simulink model "lab_2"  (R2017a)
settings: Solver=ode23tb  StartTime=0.0  StopTime=10.0  RelTol=1e-3
values from neighbouring files (symbols this model uses):
  c = 0.05    [K_Gain_matrix.m]    (also in Stepper_Model_2017_10_31_Script.m = 0.017; Stepper_Model_2017_Mark_Script.m)
  g = 9.82    [Stepper_Model_2017_10_31_Script.m]    (also in Stepper_Model_2017_Mark_Script.m)
  m = 0.2    [K_Gain_matrix.m]    (also in Stepper_Model_2017_10_31_Script.m; Stepper_Model_2017_Mark_Script.m)
undefined symbols (not defined in the file or in its folder): l
settings Model: Creator=c3204612  LastModifiedBy=Administrator
settings OptimizationCC: LifeSpan=inf
settings DebuggingCC: SFExecutionAtInitializationDiag=none

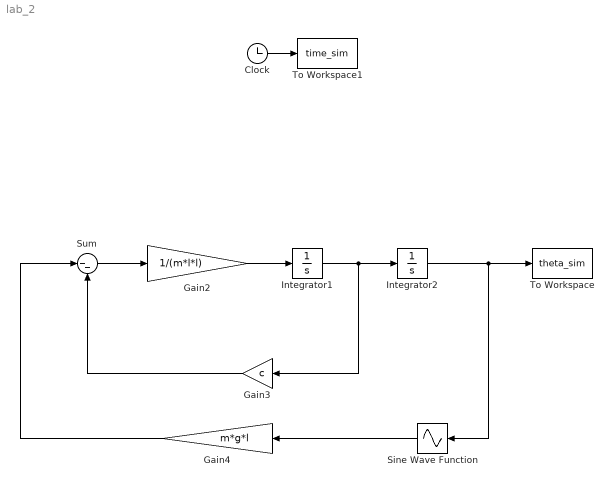
== system lab_2 ==
  Clock : Clock
  Gain2 : Gain  Gain=1/(m*l*l)
  Gain3 : Gain  Gain=c
  Gain4 : Gain  Gain=m*g*l
  Integrator1 : Integrator
  Integrator2 : Integrator
  Sine Wave Function : Sin  TimeSource=Use external signal  SampleTime=0
  Sum : Sum  Inputs=|--
  To Workspace : ToWorkspace  VariableName=theta_sim  SampleTime=-1
  To Workspace1 : ToWorkspace  VariableName=time_sim  SampleTime=-1
  wires:
  Gain4/1 -> Sum/1
  Integrator2/1 -> To Workspace/1, Sine Wave Function/1
  Gain3/1 -> Sum/2
  Sine Wave Function/1 -> Gain4/1
  Gain2/1 -> Integrator1/1
  Sum/1 -> Gain2/1
  Integrator1/1 -> Gain3/1, Integrator2/1
  Clock/1 -> To Workspace1/1
